simulink model "gm_commhdlQPSKTxRx"  (R2025b)
settings: Solver=VariableStepAuto  StartTime=0.0  StopTime=10.0  RelTol=1e-3
PostLoadFcn:
  | hScopeConfig = get_param([gcs '/Receiver/QPSK Rx/Frequency and Time Synchronizer/Symbol Synchronizer/No HDL/QPSK Receiver Eye Diagram'],'ScopeConfiguration');
  | 
  | hScopeConfig.OpenAtSimulationStart = false;
  | hScopeConfig.Visible = false;
  | SamplesPerSymbol = 4;
  | %UpsamplesRx = 1;
  | clear hScopeConfig
InitFcn:
  | commhdlQPSKTxRxModelInit;
  | % Rate bridge: ADRV9002/Jupiter radio runs at 15.36 MHz = 2x the 7.68 MHz
  | % (4 samples/symbol @ Rsym=1.92 MHz) the QPSK Rx requires. The deployed
  | % Receiver must downsample the ADC stream by 2. UpsamplesRx=1 fed the QPSK
  | % Rx 8 sps (2x-upsampled) and broke symbol sync / the loopback bit check.
  | UpsamplesRx = 2;
  | UpsamplesTx = 1;
  | clear simTimingOffset;
StopFcn:
  | if exist('simTimingOffset','var')
  |   disp('Simulation completed');
  |   %QPSKTxRxVerification;
  | end
undefined symbols (not defined in the file or in its folder): Add, Config, Error, fsym, Ignore, randsrc, RandStream, Rsym, Shift
libraries: hdlsllib x64, dspsigops x19, simulink x19, dsphdlfiltering2 x3, dsphdlsigops2 x2, dsphdlmathfun2 x2, commdigbbndpm3 x2, commchan3 x1, commrflib2 x1
(part 8 of 9)

== system gm_commhdlQPSKTxRx/Receiver/QPSK Rx/Frequency and Time Synchronizer/Phase Ambiguity Estimation and Correction/Phase Ambiguity Estimator ==
  dataIn : Inport  OutDataTypeStr=fixdt(1, 16, 14)  PortDimensions=1  SampleTime=1.30208333333333e-07
      settings: SignalType=complex
  syncPulse : Inport  Port=2  OutDataTypeStr=boolean  PortDimensions=1  SampleTime=1.30208333333333e-07
  validIn : Inport  Port=3  OutDataTypeStr=boolean  PortDimensions=1  SampleTime=1.30208333333333e-07
  Compare To Constant : simulink/Logic and Bit Operations/Compare To Constant  relop===  const=7  OutDataTypeStr=boolean
  Delay{1..3,8} (4 alike) : Delay  DelayLength=1
  Delay{4..7,9..11} (7 alike) : Delay
  Direct Lookup Table (n-D) : LookupNDDirect  NumberOfTableDimensions=1  Table=fi(preambleSymbols(3+1:3+8),1,16)  DiagnosticForOutOfRangeInput=Error
  HDL Counter : hdlsllib/Sources/HDL Counter  CountType=Count limited  CountInit=0  CountStep=1  CountMax=8-1  CountFromType=Initial value  CountFrom=0  CountResetPort=on  CountLoadPort=off  CountEnbPort=on  CountDirPort=off  CountHitOutputPort=off  CountDataType=Unsigned  CountWordLen=3  CountFracLen=0  CountSampTime=1
  Logical Operator : Logic  IconShape=distinctive  AllPortsSameDT=off  OutDataTypeStr=boolean
  Math Function : Math  Operator=conj  SignedPower=on  OutDataTypeStr=fixdt(1, 16, 15)  RndMeth=Zero
  Product : Product  OutDataTypeStr=fixdt(1, 32, 29)
  Subsystem : Subsystem
  Subsystem1 : Subsystem
  endOut : Outport  SampleTime=1.30208333333333e-07
  estOut : Outport  Port=2  SampleTime=1.30208333333333e-07
  validOut : Outport  Port=3  SampleTime=1.30208333333333e-07
  wires:
  Product/1 -> Delay9/1
  Delay11/1 -> endOut/1
  Delay5/1 -> Product/1
  Math Function/1 -> Delay4/1
  Delay1/1 -> Delay5/1
  Subsystem1/1(validOut) -> Delay2/1, Logical Operator/1, HDL Counter/2
  validIn/1 -> Subsystem1/2(validIn)
  Delay2/1 -> Delay6/1
  Subsystem/1(Out2) -> HDL Counter/1, Subsystem1/1(In1)
  Logical Operator/1 -> Delay3/1, Subsystem/2(H)
  Delay6/1 -> Delay10/1
  HDL Counter/1 -> Delay8/1, Compare To Constant/1
  Delay9/1 -> estOut/1
  Compare To Constant/1 -> Logical Operator/2
  Delay4/1 -> Product/2
  Delay10/1 -> validOut/1
  Delay3/1 -> Delay7/1
  syncPulse/1 -> Subsystem/1(L)
  Delay8/1 -> Direct Lookup Table (n-D)/1
  Delay7/1 -> Delay11/1
  dataIn/1 -> Delay1/1
  Direct Lookup Table (n-D)/1 -> Math Function/1

== system gm_commhdlQPSKTxRx/Receiver/QPSK Rx/Frequency and Time Synchronizer/Preamble Detector/Correlator ==
  dataIn : Inport  OutDataTypeStr=fixdt(1, 16, 14)  PortDimensions=1  SampleTime=1.30208333333333e-07
      settings: SignalType=complex
  validIn : Inport  Port=2  OutDataTypeStr=boolean  PortDimensions=1  SampleTime=1.30208333333333e-07
  Complex to Real-Imag : ComplexToRealImag  Output=Real
  Delay{1..6} (6 alike) : Delay  DelayLength=1
  Delay7 : Delay  DelayLength=4
  Delay8 : Delay  DelayLength=4
  Discrete FIR Filter : dsphdlfiltering2/Discrete FIR Filter  NumeratorSource=Property  Numerator=rxPreambleMFCoeffs  NumeratorPrototype=[]  FilterStructure=Direct form systolic  SerializationOption=Minimum number of cycles between valid input samples  NumCycles=2  NumberOfMultipliers=2  SimulateUsing=Code generation  roundingMode=Floor  overflowMode=off  CoefficientsDataTypeStr=Inherit: Same word length as input  OutputDataTypeStr=Inherit: Same word length as input  ResetInputPort=off  HDLGlobalReset=off  CoeffMultiplier=Multiplier  UseMultForPow2Coeff=on  FrameInputSymmOptim=off
  Magnitude Squared : Subsystem
  Magnitude Squared and Moving Sum : Subsystem
  ThresholdLimiter : Subsystem
  dataOut : Outport  SampleTime=1.30208333333333e-07
  threshold : Outport  Port=2  SampleTime=1.30208333333333e-07
  validOut : Outport  Port=3  SampleTime=1.30208333333333e-07
  wires:
  Delay2/1 -> dataOut/1
  Delay5/1 -> threshold/1
  Delay8/1 -> Delay5/1
  Delay7/1 -> Delay3/1
  validIn/1 -> Discrete FIR Filter/2, Magnitude Squared and Moving Sum/2(validIn)
  ThresholdLimiter/1(y) -> Delay8/1
  Discrete FIR Filter/1 -> Delay6/1
  Delay6/1 -> Magnitude Squared/1(In1)
  dataIn/1 -> Discrete FIR Filter/1, Magnitude Squared and Moving Sum/1(scaled1)
  Delay3/1 -> validOut/1
  Magnitude Squared and Moving Sum/1(E1) -> Delay4/1
  Discrete FIR Filter/2 -> Delay1/1
  Delay1/1 -> Delay7/1
  Delay4/1 -> ThresholdLimiter/1(x)
  Magnitude Squared/1(Out1) -> Complex to Real-Imag/1
  Complex to Real-Imag/1 -> Delay2/1

== system gm_commhdlQPSKTxRx/Receiver/QPSK Rx/Frequency and Time Synchronizer/Preamble Detector/FIFO ==
  in : Inport  OutDataTypeStr=fixdt(1, 16, 14)  PortDimensions=1  SampleTime=1.30208333333333e-07
      settings: SignalType=complex
  push : Inport  Port=2  OutDataTypeStr=boolean  PortDimensions=1  SampleTime=1.30208333333333e-07
  pop : Inport  Port=3  OutDataTypeStr=boolean  PortDimensions=1  SampleTime=1.30208333333333e-07
  reset : Inport  Port=4  OutDataTypeStr=boolean  PortDimensions=1  SampleTime=1.30208333333333e-07
  Delay1 : Delay  DelayLength=1
  Pop Counter : hdlsllib/Sources/HDL Counter  CountType=Count limited  CountInit=0  CountStep=1  CountMax=fifoSize -1  CountFromType=Initial value  CountFrom=0  CountResetPort=on  CountLoadPort=off  CountEnbPort=on  CountDirPort=off  CountHitOutputPort=off  CountDataType=Unsigned  CountWordLen=nextpow2(fifoSize)  CountFracLen=0  CountSampTime=1
  Push Counter : hdlsllib/Sources/HDL Counter  CountType=Count limited  CountInit=0  CountStep=1  CountMax=fifoSize -1  CountFromType=Initial value  CountFrom=0  CountResetPort=on  CountLoadPort=off  CountEnbPort=on  CountDirPort=off  CountHitOutputPort=off  CountDataType=Unsigned  CountWordLen=nextpow2(fifoSize)  CountFracLen=0  CountSampTime=1
  Simple Dual Port RAM : hdlsllib/HDL RAMs/Simple Dual Port RAM  ram_size=nextpow2(fifoSize)
  Validate Input Push Pop : Subsystem
  out : Outport  SampleTime=1.30208333333333e-07
  wires:
  Simple Dual Port RAM/1 -> out/1
  Pop Counter/1 -> Simple Dual Port RAM/4
  Push Counter/1 -> Simple Dual Port RAM/2
  in/1 -> Simple Dual Port RAM/1
  Delay1/1 -> Push Counter/1, Pop Counter/1
  pop/1 -> Validate Input Push Pop/3(pop)
  Validate Input Push Pop/2(valid pop) -> Pop Counter/2
  Validate Input Push Pop/1(valid push) -> Push Counter/2, Simple Dual Port RAM/3
  push/1 -> Validate Input Push Pop/2(push)
  reset/1 -> Validate Input Push Pop/1(rst), Delay1/1

== system gm_commhdlQPSKTxRx/Receiver/QPSK Rx/Frequency and Time Synchronizer/Preamble Detector/Peak Search ==
  note: peak picker
  corr : Inport  OutDataTypeStr=fixdt(1, 32, 26)  PortDimensions=1  SampleTime=1.30208333333333e-07
  thresholdExceeded : Inport  Port=2  OutDataTypeStr=boolean  PortDimensions=1  SampleTime=1.30208333333333e-07
  validIn : Inport  Port=3  OutDataTypeStr=boolean  PortDimensions=1  SampleTime=1.30208333333333e-07
  Compare To Constant : simulink/Logic and Bit Operations/Compare To Constant  relop===  const=samplesPerFrame1x - 1  OutDataTypeStr=boolean
  Logical Operator : Logic  IconShape=distinctive  AllPortsSameDT=off  OutDataTypeStr=boolean
  Logical Operator4 : Logic  IconShape=distinctive  AllPortsSameDT=off  OutDataTypeStr=boolean
  Relational Operator : RelationalOperator  Operator=>  OutDataTypeStr=boolean  InputSameDT=off
  Unit Delay Enabled Resettable Synchronous : hdlsllib/Discrete/Unit Delay Enabled Resettable Synchronous  InitialCondition=0.0  SampleTime=-1
  Unit Delay Enabled Resettable Synchronous1 : hdlsllib/Discrete/Unit Delay Enabled Resettable Synchronous  InitialCondition=0.0  SampleTime=-1
  Unit Delay Enabled Synchronous : hdlsllib/Discrete/Unit Delay Enabled Synchronous  InitialCondition=0.0  SampleTime=-1
  timing Reference : hdlsllib/Sources/HDL Counter  CountType=Count limited  CountInit=0  CountStep=1  CountMax=samplesPerFrame1x - 1  CountFromType=Initial value  CountFrom=0  CountResetPort=off  CountLoadPort=off  CountEnbPort=on  CountDirPort=off  CountHitOutputPort=off  CountDataType=Unsigned  CountWordLen=nextpow2(samplesPerFrame1x - 1)  CountFracLen=0  CountSampTime=1
  timingOffset : Outport  SampleTime=1.30208333333333e-07
  done : Outport  Port=2  SampleTime=1.30208333333333e-07
  success : Outport  Port=3  SampleTime=1.30208333333333e-07
  wires:
  Unit Delay Enabled Synchronous/1 -> timingOffset/1
  Logical Operator4/1 -> Unit Delay Enabled Synchronous/2, Unit Delay Enabled Resettable Synchronous/2
  Relational Operator/1 -> Logical Operator4/1
  Unit Delay Enabled Resettable Synchronous1/1 -> success/1
  Unit Delay Enabled Resettable Synchronous/1 -> Relational Operator/2
  corr/1 -> Unit Delay Enabled Resettable Synchronous/1, Relational Operator/1
  thresholdExceeded/1 -> Unit Delay Enabled Resettable Synchronous1/1, Unit Delay Enabled Resettable Synchronous1/2, Logical Operator4/2
  Logical Operator/1 -> done/1, Unit Delay Enabled Resettable Synchronous/3, Unit Delay Enabled Resettable Synchronous1/3
  Compare To Constant/1 -> Logical Operator/2
  timing Reference/1 -> Compare To Constant/1, Unit Delay Enabled Synchronous/1
  validIn/1 -> timing Reference/1, Logical Operator/1

== system gm_commhdlQPSKTxRx/Receiver/QPSK Rx/Frequency and Time Synchronizer/Preamble Detector/Timing Adjust ==
  timingOffset : Inport  OutDataTypeStr=fixdt(0, 11, 0)  PortDimensions=1  SampleTime=1.30208333333333e-07
  timingOffsetValid : Inport  Port=2  OutDataTypeStr=boolean  PortDimensions=1  SampleTime=1.30208333333333e-07
  dataIn : Inport  Port=3  OutDataTypeStr=fixdt(1, 16, 14)  PortDimensions=1  SampleTime=1.30208333333333e-07
      settings: SignalType=complex
  validIn : Inport  Port=4  OutDataTypeStr=boolean  PortDimensions=1  SampleTime=1.30208333333333e-07
  Delay{,1..4} (5 alike) : Delay  DelayLength=1
  Logical Operator : Logic  AllPortsSameDT=off  OutDataTypeStr=boolean
  Logical Operator1 : Logic  Operator=NOT  AllPortsSameDT=off  OutDataTypeStr=boolean
  Logical Operator2 : Logic  Inputs=3  AllPortsSameDT=off  OutDataTypeStr=boolean
  Relational Operator : RelationalOperator  Operator===  OutDataTypeStr=boolean  InputSameDT=off
  State Register : hdlsllib/Discrete/Unit Delay Enabled Resettable Synchronous  InitialCondition=0.0  SampleTime=-1
  Unit Delay Enabled Synchronous3 : hdlsllib/Discrete/Unit Delay Enabled Synchronous  InitialCondition=0.0  SampleTime=-1
  timing Reference : hdlsllib/Sources/HDL Counter  CountType=Count limited  CountInit=0  CountStep=1  CountMax=searchSamples - 1  CountFromType=Initial value  CountFrom=0  CountResetPort=off  CountLoadPort=off  CountEnbPort=on  CountDirPort=off  CountHitOutputPort=off  CountDataType=Unsigned  CountWordLen=nextpow2(searchSamples - 1)  CountFracLen=0  CountSampTime=1
  dataOut : Outport  SampleTime=1.30208333333333e-07
  validOut : Outport  Port=2  SampleTime=1.30208333333333e-07
  SyncPulse : Outport  Port=3  SampleTime=1.30208333333333e-07
  wires:
  Delay/1 -> SyncPulse/1
  Logical Operator2/1 -> Delay/1, Delay2/1
  timingOffsetValid/1 -> Logical Operator/1
  dataIn/1 -> Delay4/1
  Logical Operator1/1 -> Logical Operator/2
  Delay4/1 -> dataOut/1
  validIn/1 -> timing Reference/1, Delay3/1, Logical Operator2/1
  timingOffset/1 -> Unit Delay Enabled Synchronous3/1
  Logical Operator/1 -> State Register/1, State Register/2, Unit Delay Enabled Synchronous3/2
  Delay3/1 -> validOut/1
  Unit Delay Enabled Synchronous3/1 -> Relational Operator/2
  timing Reference/1 -> Relational Operator/1
  Relational Operator/1 -> Logical Operator2/2
  State Register/1 -> Logical Operator2/3, Delay1/1
  Delay1/1 -> Logical Operator1/1
  Delay2/1 -> State Register/3

== system gm_commhdlQPSKTxRx/Receiver/QPSK Rx/Frequency and Time Synchronizer/Symbol Synchronizer/Gardner TED ==
  data : Inport  OutDataTypeStr=fixdt(1, 19, 12)  PortDimensions=1  SampleTime=1.30208333333333e-07
      settings: SignalType=complex
  strobe : Inport  Port=2  OutDataTypeStr=boolean  PortDimensions=1  SampleTime=1.30208333333333e-07
  Constant : Constant  Value=0  OutDataTypeStr=fixdt(1, 40, 24)  SampleTime=1/(Rsym*SamplesPerSymbol)
  Delay10 : Delay  DelayLength=4
  GTED : Subsystem
  Switch : Switch  Criteria=u2 ~= 0  OutDataTypeStr=fixdt(1, 40, 24)  InputSameDT=off
  e : Outport  SampleTime=1.30208333333333e-07  VectorParamsAs1DForOutWhenUnconnected=off
  wires:
  Switch/1 -> e/1
  Delay10/1 -> Switch/2
  GTED/1(Out1) -> Switch/1
  strobe/1 -> Delay10/1
  Constant/1 -> Switch/3
  data/1 -> GTED/1(In1)

== system gm_commhdlQPSKTxRx/Receiver/QPSK Rx/Frequency and Time Synchronizer/Symbol Synchronizer/Interpolation Control ==
  Delta : Inport  OutDataTypeStr=fixdt(1, 11, 10)  PortDimensions=1  SampleTime=1.30208333333333e-07
  Interpolation Control : MATLAB Function
  mu : Outport  SampleTime=1.30208333333333e-07
  Underflow : Outport  Port=2  SampleTime=1.30208333333333e-07
  wires:
  Delta/1 -> Interpolation Control/1(Delta)
  Interpolation Control/1(mu) -> mu/1
  Interpolation Control/2(Underflow) -> Underflow/1

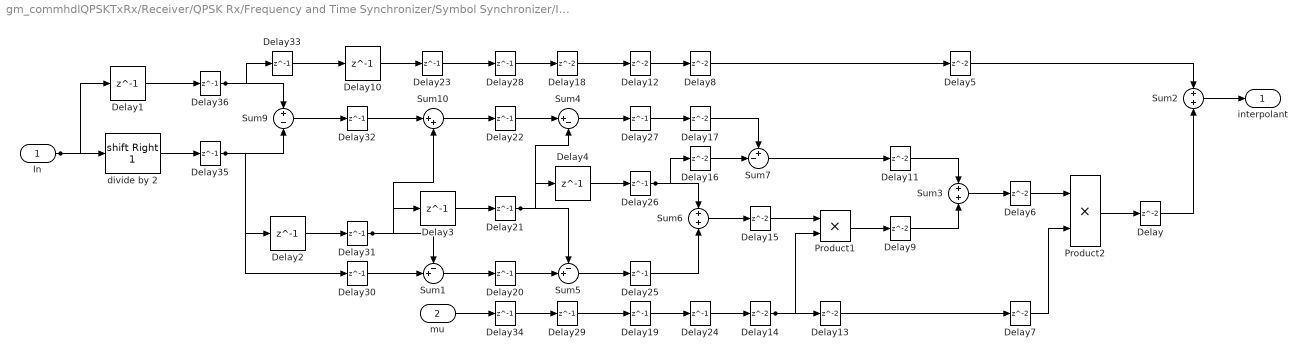
== system gm_commhdlQPSKTxRx/Receiver/QPSK Rx/Frequency and Time Synchronizer/Symbol Synchronizer/Interpolation Filter ==
  In : Inport  OutDataTypeStr=fixdt(1, 16, 12)  PortDimensions=1  SampleTime=1.30208333333333e-07
      settings: SignalType=complex
  mu : Inport  Port=2  OutDataTypeStr=fixdt(1, 11, 10)  PortDimensions=1  SampleTime=1.30208333333333e-07
  Delay{,5..9,11..18} (14 alike) : Delay
  Delay{1..4,10} (5 alike) : Delay  DelayLength=1  InitialCondition=0
  Delay{19..36} (18 alike) : Delay  DelayLength=1
  Product1 : Product  OutDataTypeStr=fixdt(1,16,10)  RndMeth=Zero
  Product2 : Product  OutDataTypeStr=fixdt(1, 16, 10)  RndMeth=Zero
  Sum1 : Sum  Inputs=-+|  OutDataTypeStr=fixdt(1, 17, 12)
  Sum10 : Sum  Inputs=|++  OutDataTypeStr=fixdt(1, 18, 12)
  Sum2 : Sum  Inputs=+|+  OutDataTypeStr=fixdt(1, 19, 12)
  Sum3 : Sum  Inputs=+|+  OutDataTypeStr=fixdt(1,16,10)
  Sum4 : Sum  Inputs=|+-  OutDataTypeStr=fixdt(1, 19, 12)
  Sum5 : Sum  Inputs=-+|  OutDataTypeStr=fixdt(1, 18, 12)
  Sum6 : Sum  Inputs=+|+  OutDataTypeStr=fixdt(1,16,11)  SaturateOnIntegerOverflow=on
  Sum7 : Sum  Inputs=+-|  OutDataTypeStr=fixdt(1,16,10)
  Sum9 : Sum  Inputs=+-  OutDataTypeStr=fixdt(1, 17, 12)
  divide by 2 : ArithShift  BitShiftNumber=1  BitShiftDirection=Right
  interpolant : Outport  SampleTime=1.30208333333333e-07
  wires:
  Delay/1 -> Sum2/2
  Product2/1 -> Delay/1
  Delay6/1 -> Product2/1
  Delay5/1 -> Sum2/1
  Delay13/1 -> Delay7/1
  Sum7/1 -> Delay11/1
  Sum3/1 -> Delay6/1
  Delay24/1 -> Delay14/1
  Delay16/1 -> Sum7/2
  Delay17/1 -> Sum7/1
  Delay8/1 -> Delay5/1
  Delay19/1 -> Delay24/1
  Delay26/1 -> Delay16/1, Sum6/1
  Delay7/1 -> Product2/2
  Delay31/1 -> Delay3/1, Sum1/1, Sum10/2
  Delay15/1 -> Product1/1
  Delay2/1 -> Delay31/1
  Delay35/1 -> Delay2/1, Delay30/1, Sum9/2
  Sum9/1 -> Delay32/1
  Delay23/1 -> Delay28/1
  Sum1/1 -> Delay20/1
  Delay33/1 -> Delay10/1
  Delay4/1 -> Delay26/1
  Delay36/1 -> Delay33/1, Sum9/1
  Delay25/1 -> Sum6/2
  Delay12/1 -> Delay8/1
  Sum5/1 -> Delay25/1
  Delay28/1 -> Delay18/1
  divide by 2/1 -> Delay35/1
  Delay1/1 -> Delay36/1
  Delay14/1 -> Delay13/1, Product1/2
  Delay3/1 -> Delay21/1
  Product1/1 -> Delay9/1
  Delay34/1 -> Delay29/1
  Delay30/1 -> Sum1/2
  Delay32/1 -> Sum10/1
  Delay10/1 -> Delay23/1
  Sum4/1 -> Delay27/1
  Sum10/1 -> Delay22/1
  Delay9/1 -> Sum3/2
  Delay21/1 -> Delay4/1, Sum4/2, Sum5/1
  Delay11/1 -> Sum3/1
  mu/1 -> Delay34/1
  Sum2/1 -> interpolant/1
  In/1 -> Delay1/1, divide by 2/1
  Delay22/1 -> Sum4/1
  Delay20/1 -> Sum5/2
  Delay18/1 -> Delay12/1
  Delay29/1 -> Delay19/1
  Sum6/1 -> Delay15/1
  Delay27/1 -> Delay17/1

== system gm_commhdlQPSKTxRx/Receiver/QPSK Rx/Frequency and Time Synchronizer/Symbol Synchronizer/Loop Filter ==
  e : Inport  OutDataTypeStr=fixdt(1, 40, 24)  PortDimensions=1  SampleTime=1.30208333333333e-07
  Add : Sum  OutDataTypeStr=fixdt(1, 31, 23)
  Add2 : Sum  Inputs=|++  OutDataTypeStr=fixdt(1, 30, 23)
  Data Type Conversion17 : DataTypeConversion  OutDataTypeStr=fixdt(1,11,10)  SaturateOnIntegerOverflow=off  RndMeth=Floor
  Delay : Delay  DelayLength=1
  Delay1 : Delay  DelayLength=1  InitialCondition=0
  Delay2 : Delay  InitialCondition=0
  Delay3 : Delay  InitialCondition=0
  Delay4 : Delay  DelayLength=1  InitialCondition=0
  Delay5 : Delay  InitialCondition=0
  Delay6 : Delay  DelayLength=1
  K1 : Gain  Gain=fi(SSLoopFilterPropGain,1,24,24)  ParamDataTypeStr=Inherit: Inherit from 'Gain'  OutDataTypeStr=fixdt(1,30,23)
  K2 : Gain  Gain=fi(SSLoopFilterIntegGain,1,24,24)  ParamDataTypeStr=Inherit: Inherit from 'Gain'  OutDataTypeStr=fixdt(1,30,23)
  v : Outport  SampleTime=1.30208333333333e-07
  wires:
  Add2/1 -> Delay4/1, Delay/1
  Delay6/1 -> Add2/1
  Add/1 -> Data Type Conversion17/1
  Delay/1 -> Add2/2
  Delay5/1 -> Delay6/1
  Data Type Conversion17/1 -> v/1
  Delay4/1 -> Add/2
  Delay3/1 -> Delay1/1
  K2/1 -> Delay5/1
  K1/1 -> Delay3/1
  Delay1/1 -> Add/1
  Delay2/1 -> K1/1, K2/1
  e/1 -> Delay2/1

== system gm_commhdlQPSKTxRx/Receiver/QPSK Rx/Frequency and Time Synchronizer/Symbol Synchronizer/Rate Handle ==
  dataIn : Inport  OutDataTypeStr=fixdt(1, 16, 14)  PortDimensions=1  SampleTime=1.30208333333333e-07
      settings: SignalType=complex
  strobe : Inport  Port=2  OutDataTypeStr=boolean  PortDimensions=1  SampleTime=1.30208333333333e-07
  validIn : Inport  Port=3  OutDataTypeStr=boolean  PortDimensions=1  SampleTime=1.30208333333333e-07
  Compare To Constant : simulink/Logic and Bit Operations/Compare To Constant  relop===  const=0  OutDataTypeStr=boolean
  Constant : Constant  Value=false  OutDataTypeStr=boolean  SampleTime=-1
  FIFO : Subsystem  mask{fifoSize=double(32), pushFullDiag=Error, popEmptyDiag=Ignore}
      mask prompts: fifoSize "FIFO size:"; pushFullDiag "Push full FIFO:"; popEmptyDiag "Pop empty FIFO:"
      mask TypeOptions pushFullDiag: Ignore | Warning | Error
      mask TypeOptions popEmptyDiag: Ignore | Warning | Error
  HDL Counter : hdlsllib/Sources/HDL Counter  CountType=Count limited  CountInit=0  CountStep=1  CountMax=SamplesPerSymbol - 1  CountFromType=Initial value  CountFrom=0  CountResetPort=off  CountLoadPort=off  CountEnbPort=on  CountDirPort=off  CountHitOutputPort=off  CountDataType=Unsigned  CountWordLen=nextpow2(SamplesPerSymbol - 1)  CountFracLen=0  CountSampTime=1
  Logical Operator : Logic  AllPortsSameDT=off  OutDataTypeStr=boolean
  dataOut : Outport  SampleTime=1.30208333333333e-07
  validOut : Outport  Port=2  SampleTime=1.30208333333333e-07
  wires:
  FIFO/2(validPop) -> validOut/1
  FIFO/1(out) -> dataOut/1
  strobe/1 -> FIFO/2(push)
  dataIn/1 -> FIFO/1(in)
  Logical Operator/1 -> FIFO/3(pop)
  Compare To Constant/1 -> Logical Operator/2
  Constant/1 -> FIFO/4(reset)
  HDL Counter/1 -> Compare To Constant/1
  validIn/1 -> HDL Counter/1, Logical Operator/1

== system gm_commhdlQPSKTxRx/Transmitter/QPSK Tx/Bit Packetizer/Data Bits FIFO/No HDL ==
  push : Inport
  pop : Inport  Port=2
  MATLAB Function : MATLAB Function  TreatAsAtomicUnit=on
  No HDL : Subsystem
  wires:
  MATLAB Function/3(empty) -> No HDL/4(empty)
  MATLAB Function/1(full) -> No HDL/2(full)
  MATLAB Function/2(ncount) -> No HDL/3(ncount)
  pop/1 -> No HDL/5(pop), MATLAB Function/2(rd)
  push/1 -> No HDL/1(push), MATLAB Function/1(wr)

== system gm_commhdlQPSKTxRx/Transmitter/QPSK Tx/Bit Packetizer/Preamble Bits Generator/Preamble Bits Store ==
  note: The Preamble is padded with zeros in the LUT such that
      | the length is the 2^nextpow2(length(Preamble)) for
      | efficient resource mapping to RAM
  actualPreamble : Inport
  sampleCount : Inport  Port=2
  Constant : Constant  OutDataTypeStr=boolean  SampleTime=1/(Rsym*4)
  Extract Bits : simulink/Logic and Bit Operations/Extract Bits  bitsToExtract=Range of bits  numBits=8  bitIdxRange=[0 nextpow2(length(Preamble))-1]  outScalingMode=Treat bit field as an integer
  Preamble : LookupNDDirect  NumberOfTableDimensions=1  Table=[Preamble;false(32-length(Preamble),1)]  DiagnosticForOutOfRangeInput=Error
  Switch : Switch  Criteria=u2 ~= 0  Threshold=1  SaturateOnIntegerOverflow=off  InputSameDT=off
  preamble : Outport
  wires:
  actualPreamble/1 -> Switch/2
  sampleCount/1 -> Extract Bits/1
  Preamble/1 -> Switch/1
  Extract Bits/1 -> Preamble/1
  Constant/1 -> Switch/3
  Switch/1 -> preamble/1

== system gm_commhdlQPSKTxRx/Receiver/QPSK Rx/Frequency and Time Synchronizer/Coarse Frequency Compensator/Coarse Frequency Estimator/Extract Frequency ==
  datain : Inport  OutDataTypeStr=fixdt(1, 32, 24)  PortDimensions=1  SampleTime=1.30208333333333e-07
      settings: SignalType=complex
  validIn : Inport  Port=2  OutDataTypeStr=boolean  PortDimensions=1  SampleTime=1.30208333333333e-07
  Complex to Magnitude-Angle HDL Optimized : dsphdlmathfun2/Complex to Magnitude-Angle  NumIterationsSource=Auto  NumIterations=10  OutputFormat=Angle  AngleFormat=Normalized  ScaleOutput=on  ScalingMethod=Shift-Add  SimulateUsing=Code generation
  Delay{1..4} (4 alike) : Delay  DelayLength=1
  Gain : Gain  Gain=1/2  ParamDataTypeStr=fixdt(0,1,1)  OutDataTypeStr=fixdt(1, 35, 34)
  Unit Delay Enabled Synchronous : hdlsllib/Discrete/Unit Delay Enabled Synchronous  InitialCondition=0.0  SampleTime=-1
  normFreqOut : Outport  SampleTime=1.30208333333333e-07
  wires:
  Delay3/1 -> normFreqOut/1
  Gain/1 -> Delay3/1
  Delay2/1 -> Gain/1
  Unit Delay Enabled Synchronous/1 -> Delay2/1
  Complex to Magnitude-Angle HDL Optimized/2 -> Unit Delay Enabled Synchronous/2
  Complex to Magnitude-Angle HDL Optimized/1 -> Unit Delay Enabled Synchronous/1
  Delay4/1 -> Complex to Magnitude-Angle HDL Optimized/2
  Delay1/1 -> Complex to Magnitude-Angle HDL Optimized/1
  validIn/1 -> Delay4/1
  datain/1 -> Delay1/1

== system gm_commhdlQPSKTxRx/Receiver/QPSK Rx/Frequency and Time Synchronizer/Coarse Frequency Compensator/Coarse Frequency Estimator/Integrator ==
  note: store the value in the Reg before reset
  dataIn : Inport  OutDataTypeStr=fixdt(1, 32, 24)  PortDimensions=1  SampleTime=1.30208333333333e-07
      settings: SignalType=complex
  validIn : Inport  Port=2  OutDataTypeStr=boolean  PortDimensions=1  SampleTime=1.30208333333333e-07
  Add1 : Sum  Inputs=|++  OutDataTypeStr=fixdt(1, 32, 24)
  Delay : Delay  DelayLength=1
  Delay1 : Delay  DelayLength=1
  Delay2 : Delay  DelayLength=1
  Integ Reg : hdlsllib/Discrete/Unit Delay Enabled Resettable Synchronous  InitialCondition=0.0  SampleTime=-1
  Reset Generator : Subsystem
  Store Reg : hdlsllib/Discrete/Unit Delay Enabled Synchronous  InitialCondition=0.0  SampleTime=-1
  IntegOut : Outport  SampleTime=1.30208333333333e-07
  IntegValid : Outport  Port=2  SampleTime=1.30208333333333e-07
  wires:
  Add1/1 -> Integ Reg/1
  Integ Reg/1 -> Store Reg/1, Add1/2
  Delay1/1 -> Add1/1
  Delay/1 -> IntegValid/1
  Delay2/1 -> Integ Reg/2
  dataIn/1 -> Delay1/1
  Store Reg/1 -> IntegOut/1
  Reset Generator/1(reset) -> Delay/1, Integ Reg/3, Store Reg/2
  validIn/1 -> Reset Generator/1(validIn), Delay2/1

== system gm_commhdlQPSKTxRx/Receiver/QPSK Rx/Frequency and Time Synchronizer/Phase Ambiguity Estimation and Correction/Phase Ambiguity Corrector/Reciprocal ==
  dataIn : Inport  OutDataTypeStr=fixdt(1, 13, 10)  PortDimensions=1  SampleTime=1.30208333333333e-07
  Compare To Constant : simulink/Logic and Bit Operations/Compare To Constant  relop=<  const=0  OutDataTypeStr=boolean
  Data Type Conversion : DataTypeConversion  OutDataTypeStr=fixdt(1,WL,0)  ConvertRealWorld=Stored Integer (SI)  SaturateOnIntegerOverflow=off  RndMeth=Floor
  Data Type Conversion1 : DataTypeConversion  OutDataTypeStr=fixdt(0,LUTAddrWL,0)  ConvertRealWorld=Stored Integer (SI)  SaturateOnIntegerOverflow=off  RndMeth=Floor
  Data Type Conversion2 : DataTypeConversion  OutDataTypeStr=fixdt(0,WL-LUTAddrWL,0)  ConvertRealWorld=Stored Integer (SI)  SaturateOnIntegerOverflow=off  RndMeth=Floor
  Delay : Delay  DelayLength=1
  Delay1 : Delay  DelayLength=1
  Delay2 : Delay  DelayLength=1
  Extract Bits : simulink/Logic and Bit Operations/Extract Bits  bitsToExtract=Range ending with least significant bit  numBits=LUTAddrWL  bitIdxRange=[0 7]  outScalingMode=Treat bit field as an integer
  Function Impl : Subsystem
  dataOut : Outport  SampleTime=1.30208333333333e-07
  wires:
  Function Impl/1(functionValues) -> dataOut/1
  Data Type Conversion2/1 -> Function Impl/1(switch)
  Data Type Conversion1/1 -> Function Impl/2(LUTAddr)
  Delay1/1 -> Data Type Conversion2/1
  Compare To Constant/1 -> Delay1/1
  Delay2/1 -> Data Type Conversion1/1
  Extract Bits/1 -> Delay2/1
  Delay/1 -> Compare To Constant/1, Extract Bits/1
  Data Type Conversion/1 -> Delay/1
  dataIn/1 -> Data Type Conversion/1

== system gm_commhdlQPSKTxRx/Receiver/QPSK Rx/Frequency and Time Synchronizer/Phase Ambiguity Estimation and Correction/Phase Ambiguity Estimator/Subsystem ==
  L : Inport  OutDataTypeStr=boolean  PortDimensions=1  SampleTime=1.30208333333333e-07
  H : Inport  Port=2  OutDataTypeStr=boolean  PortDimensions=1  SampleTime=1.30208333333333e-07
  Delay6 : Delay  DelayLength=1  InitialCondition=1
  Logical Operator : Logic  AllPortsSameDT=off  OutDataTypeStr=boolean
  Logical Operator1 : Logic  Operator=NOT  IconShape=distinctive  AllPortsSameDT=off  OutDataTypeStr=boolean
  Logical Operator2 : Logic  Operator=OR  AllPortsSameDT=off  OutDataTypeStr=boolean
  Out2 : Outport  SampleTime=1.30208333333333e-07
  wires:
  Logical Operator/1 -> Logical Operator2/2
  Delay6/1 -> Out2/1, Logical Operator/2
  Logical Operator1/1 -> Logical Operator/1
  Logical Operator2/1 -> Delay6/1
  L/1 -> Logical Operator1/1
  H/1 -> Logical Operator2/1

== system gm_commhdlQPSKTxRx/Receiver/QPSK Rx/Frequency and Time Synchronizer/Phase Ambiguity Estimation and Correction/Phase Ambiguity Estimator/Subsystem1 ==
  In1 : Inport  OutDataTypeStr=boolean  PortDimensions=1  SampleTime=1.30208333333333e-07
  validIn : Inport  Port=2  OutDataTypeStr=boolean  PortDimensions=1  SampleTime=1.30208333333333e-07
  Logical Operator1 : Logic  IconShape=distinctive  AllPortsSameDT=off  OutDataTypeStr=boolean
  Logical Operator2 : Logic  Operator=NOT  IconShape=distinctive  AllPortsSameDT=off  OutDataTypeStr=boolean
  validOut : Outport  SampleTime=1.30208333333333e-07
  wires:
  Logical Operator1/1 -> validOut/1
  validIn/1 -> Logical Operator1/2
  Logical Operator2/1 -> Logical Operator1/1
  In1/1 -> Logical Operator2/1

== system gm_commhdlQPSKTxRx/Receiver/QPSK Rx/Frequency and Time Synchronizer/Preamble Detector/Correlator/Magnitude Squared ==
  In1 : Inport  OutDataTypeStr=fixdt(1, 16, 13)  PortDimensions=1  SampleTime=1.30208333333333e-07
      settings: SignalType=complex
  Delay1 : Delay
  Delay2 : Delay
  Delay3 : Delay
  Math Function : Math  Operator=conj  OutDataTypeStr=fixdt(1, 16, 13)
  Product : Product  OutDataTypeStr=fixdt(1, 32, 26)
  Out1 : Outport  SampleTime=1.30208333333333e-07
  wires:
  Delay1/1 -> Product/2
  Delay2/1 -> Product/1
  Math Function/1 -> Delay1/1
  Delay3/1 -> Out1/1
  Product/1 -> Delay3/1
  In1/1 -> Math Function/1, Delay2/1

== system gm_commhdlQPSKTxRx/Receiver/QPSK Rx/Frequency and Time Synchronizer/Preamble Detector/Correlator/Magnitude Squared and Moving Sum ==
  scaled1 : Inport  OutDataTypeStr=fixdt(1, 16, 14)  PortDimensions=1  SampleTime=1.30208333333333e-07
      settings: SignalType=complex
  validIn : Inport  Port=2  OutDataTypeStr=boolean  PortDimensions=1  SampleTime=1.30208333333333e-07
  Add : Sum  Inputs=|+-  OutDataTypeStr=fixdt(1, 32, 28)
  Add1 : Sum  Inputs=|++  OutDataTypeStr=fixdt(1, 32, 28)
  Complex to Real-Imag1 : ComplexToRealImag  Output=Real
  Delay : Delay  DelayLength=13  ShowEnablePort=on
      settings: InputPortMap=u0,e6
  Delay{1..4,6,8..10,12} (9 alike) : Delay
  Delay11 : Delay  DelayLength=11
  Delay14 : Delay  DelayLength=1  ShowEnablePort=on
      settings: InputPortMap=u0,e6
  Delay5 : Delay  DelayLength=1
  Delay7 : Delay  DelayLength=1
  Gain : Gain  Gain=ThresoldGainFac  OutDataTypeStr=fixdt(1, 32, 28)
  Math Function1 : Math  Operator=conj  OutDataTypeStr=fixdt(1, 16, 14)
  Product1 : Product  OutDataTypeStr=fixdt(1, 32, 28)
  E1 : Outport  SampleTime=1.30208333333333e-07
  wires:
  Delay5/1 -> Add1/1
  Add/1 -> Delay5/1
  Delay/1 -> Add/2
  Delay8/1 -> Delay/2, Delay7/1
  Delay11/1 -> E1/1
  Delay7/1 -> Delay14/2
  Delay4/1 -> Delay/1, Add/1
  scaled1/1 -> Math Function1/1, Delay6/1
  Delay6/1 -> Product1/1
  Delay14/1 -> Add1/2
  Delay3/1 -> Gain/1
  Product1/1 -> Delay2/1
  Delay1/1 -> Product1/2
  Complex to Real-Imag1/1 -> Delay3/1
  Delay2/1 -> Complex to Real-Imag1/1
  Delay12/1 -> Delay10/1
  Math Function1/1 -> Delay1/1
  validIn/1 -> Delay12/1
  Delay10/1 -> Delay9/1
  Gain/1 -> Delay4/1
  Add1/1 -> Delay11/1, Delay14/1
  Delay9/1 -> Delay8/1

== system gm_commhdlQPSKTxRx/Receiver/QPSK Rx/Frequency and Time Synchronizer/Preamble Detector/Correlator/ThresholdLimiter ==
  x : Inport  OutDataTypeStr=fixdt(1, 32, 28)  PortDimensions=1  SampleTime=1.30208333333333e-07
  ThresholdLimiter : MATLAB Function  TreatAsAtomicUnit=on
  y : Outport  SampleTime=1.30208333333333e-07  VectorParamsAs1DForOutWhenUnconnected=off
  wires:
  ThresholdLimiter/1(y) -> y/1
  x/1 -> ThresholdLimiter/1(x)

== system gm_commhdlQPSKTxRx/Receiver/QPSK Rx/Frequency and Time Synchronizer/Preamble Detector/FIFO/Validate Input Push Pop ==
  rst : Inport  OutDataTypeStr=boolean  PortDimensions=1  SampleTime=1.30208333333333e-07
  push : Inport  Port=2  OutDataTypeStr=boolean  PortDimensions=1  SampleTime=1.30208333333333e-07
  pop : Inport  Port=3  OutDataTypeStr=boolean  PortDimensions=1  SampleTime=1.30208333333333e-07
  Compare To Constant : Subsystem  mask(Compare To Constant){relop===, const=double(0), OutDataTypeStr=boolean, ZeroCross=on}
      mask prompts: relop "Simulink:masks:Operator_MP"; const "Simulink:masks:ConstantValue_MP"; OutDataTypeStr "Simulink:masks:OutputDataType_MP"; ZeroCross "Simulink:masks:EnableZerocrossingDetection_MP"
      mask help: Simulink:masks:CompareToConstant_MD
      mask init:
      | OutDataTypeStr = 'boolean';
      | ZeroCross = 'on';
      | blkName = 'commhdlQPSKTxRx/Receiver/QPSK Rx/Frequency and Time Synchronizer/Preamble Detector/FIFO/Validate Input Push Pop/Compare\nTo Constant';
      | const = double(0);
      | const_str = '0';
      | const_val = double(0);
      | relop = '==';
      | setValue = 'boolean';
      | str = '== 0';
      mask TypeOptions relop: == | ~= | < | <= | >= | >
      mask TypeOptions OutDataTypeStr: Simulink:masks:uint8 | Simulink:masks:boolean
      mask Callback ZeroCross: sl('zeroCrossEnable', gcbh);
      mask Display: disp(str)
  Compare To Constant1 : Subsystem  mask(Compare To Constant){relop===, const=double(1133), OutDataTypeStr=boolean, ZeroCross=on}
      mask prompts: relop "Simulink:masks:Operator_MP"; const "Simulink:masks:ConstantValue_MP"; OutDataTypeStr "Simulink:masks:OutputDataType_MP"; ZeroCross "Simulink:masks:EnableZerocrossingDetection_MP"
      mask help: Simulink:masks:CompareToConstant_MD
      mask init:
      | OutDataTypeStr = 'boolean';
      | ZeroCross = 'on';
      | blkName = 'commhdlQPSKTxRx/Receiver/QPSK Rx/Frequency and Time Synchronizer/Preamble Detector/FIFO/Validate Input Push Pop/Compare\nTo Constant1';
      | const = double(1133);
      | const_str = 'fifoSize';
      | const_val = [];
      | relop = '==';
      | setValue = 'boolean';
      | str = '== fifoSize';
      mask TypeOptions relop: == | ~= | < | <= | >= | >
      mask TypeOptions OutDataTypeStr: Simulink:masks:uint8 | Simulink:masks:boolean
      mask Callback ZeroCross: sl('zeroCrossEnable', gcbh);
      mask Display: disp(str)
  Constant : Constant  Value=true  OutDataTypeStr=boolean  SampleTime=-1
  Constant1 : Constant  Value=false  OutDataTypeStr=boolean  SampleTime=-1
  Delay : Delay  DelayLength=1
  Logical Operator1 : Logic  Operator=XOR  AllPortsSameDT=off  OutDataTypeStr=boolean
  Logical Operator2 : Logic  Operator=NOT  AllPortsSameDT=off  OutDataTypeStr=boolean
  Logical Operator{3..5,7,9} (5 alike) : Logic  AllPortsSameDT=off  OutDataTypeStr=boolean
  Logical Operator6 : Logic  Operator=NOT  AllPortsSameDT=off  OutDataTypeStr=boolean
  Logical Operator8 : Logic  Operator=NOT  AllPortsSameDT=off  OutDataTypeStr=boolean
  MATLAB Function : Subsystem
  Switch : Switch  Criteria=u2 ~= 0  OutDataTypeStr=boolean  SaturateOnIntegerOverflow=off  InputSameDT=off
  valid push : Outport  SampleTime=1.30208333333333e-07
  valid pop : Outport  Port=2  SampleTime=1.30208333333333e-07
  wires:
  Compare To Constant1/1(y) -> Logical Operator4/2
  Compare To Constant/1(y) -> Logical Operator3/1
  Delay/1 -> Compare To Constant/1(u), Compare To Constant1/1(u)
  push/1 -> Logical Operator9/1, Logical Operator5/1
  Logical Operator6/1 -> Logical Operator7/2
  pop/1 -> Logical Operator7/1, Logical Operator3/2
  Logical Operator3/1 -> Logical Operator6/1
  Logical Operator9/1 -> valid push/1, Logical Operator1/1
  rst/1 -> MATLAB Function/1(rst)
  Constant/1 -> Switch/3
  Logical Operator8/1 -> Logical Operator5/2
  Logical Operator4/1 -> Logical Operator2/1
  Constant1/1 -> Switch/1
  Logical Operator5/1 -> Logical Operator4/1
  Logical Operator7/1 -> valid pop/1, Logical Operator1/2, Switch/2, Logical Operator8/1
  Logical Operator1/1 -> MATLAB Function/2(enb)
  Switch/1 -> MATLAB Function/3(dir)
  Logical Operator2/1 -> Logical Operator9/2
  MATLAB Function/1(count) -> Delay/1

== system gm_commhdlQPSKTxRx/Receiver/QPSK Rx/Frequency and Time Synchronizer/Symbol Synchronizer/Gardner TED/GTED ==
  In1 : Inport  OutDataTypeStr=fixdt(1, 19, 12)  PortDimensions=1  SampleTime=1.30208333333333e-07
      settings: SignalType=complex
  Add : Sum  OutDataTypeStr=fixdt(1, 40, 24)
  Add1 : Sum  Inputs=+-  OutDataTypeStr=fixdt(1, 20, 12)
  Add2 : Sum  Inputs=+-  OutDataTypeStr=fixdt(1, 20, 12)
  Complex to Real-Imag : ComplexToRealImag
  Delay{,1..7} (8 alike) : Delay  DelayLength=1
  Delay{8..13} (6 alike) : Delay
  Product : Product  OutDataTypeStr=fixdt(1, 39, 24)
  Product1 : Product  OutDataTypeStr=fixdt(1, 39, 24)
  Out1 : Outport  SampleTime=1.30208333333333e-07
  wires:
  Delay13/1 -> Add/2
  Product1/1 -> Delay13/1
  Product/1 -> Delay10/1
  Delay9/1 -> Product/2
  Add2/1 -> Delay12/1
  Complex to Real-Imag/1 -> Delay/1, Add1/2
  Complex to Real-Imag/2 -> Delay4/1, Add2/2
  Add/1 -> Out1/1
  Delay10/1 -> Add/1
  Delay6/1 -> Delay7/1
  Delay/1 -> Delay1/1
  Delay7/1 -> Add2/1
  Delay4/1 -> Delay5/1
  In1/1 -> Complex to Real-Imag/1
  Delay3/1 -> Add1/1
  Delay12/1 -> Product1/2
  Delay1/1 -> Delay2/1, Delay8/1
  Delay11/1 -> Product1/1
  Delay5/1 -> Delay6/1, Delay11/1
  Delay2/1 -> Delay3/1
  Delay8/1 -> Product/1
  Add1/1 -> Delay9/1

== system gm_commhdlQPSKTxRx/Receiver/QPSK Rx/Frequency and Time Synchronizer/Symbol Synchronizer/Rate Handle/FIFO ==
  in : Inport  OutDataTypeStr=fixdt(1, 16, 14)  PortDimensions=1  SampleTime=1.30208333333333e-07
      settings: SignalType=complex
  push : Inport  Port=2  OutDataTypeStr=boolean  PortDimensions=1  SampleTime=1.30208333333333e-07
  pop : Inport  Port=3  OutDataTypeStr=boolean  PortDimensions=1  SampleTime=1.30208333333333e-07
  reset : Inport  Port=4  OutDataTypeStr=boolean  PortDimensions=1  SampleTime=1.30208333333333e-07
  Delay1 : Delay  DelayLength=1
  Pop Counter : hdlsllib/Sources/HDL Counter  CountType=Count limited  CountInit=0  CountStep=1  CountMax=fifoSize -1  CountFromType=Initial value  CountFrom=0  CountResetPort=on  CountLoadPort=off  CountEnbPort=on  CountDirPort=off  CountHitOutputPort=off  CountDataType=Unsigned  CountWordLen=nextpow2(fifoSize)  CountFracLen=0  CountSampTime=1
  Push Counter : hdlsllib/Sources/HDL Counter  CountType=Count limited  CountInit=0  CountStep=1  CountMax=fifoSize -1  CountFromType=Initial value  CountFrom=0  CountResetPort=on  CountLoadPort=off  CountEnbPort=on  CountDirPort=off  CountHitOutputPort=off  CountDataType=Unsigned  CountWordLen=nextpow2(fifoSize)  CountFracLen=0  CountSampTime=1
  Simple Dual Port RAM : hdlsllib/HDL RAMs/Simple Dual Port RAM  ram_size=nextpow2(fifoSize)
  Validate Input Push Pop : Subsystem
  out : Outport  SampleTime=1.30208333333333e-07
  validPop : Outport  Port=2  SampleTime=1.30208333333333e-07
  wires:
  Simple Dual Port RAM/1 -> out/1
  Pop Counter/1 -> Simple Dual Port RAM/4
  Validate Input Push Pop/1(valid push) -> Push Counter/2, Simple Dual Port RAM/3
  Push Counter/1 -> Simple Dual Port RAM/2
  Delay1/1 -> Push Counter/1, Pop Counter/1
  pop/1 -> Validate Input Push Pop/3(pop)
  Validate Input Push Pop/2(valid pop) -> Pop Counter/2, validPop/1
  push/1 -> Validate Input Push Pop/2(push)
  in/1 -> Simple Dual Port RAM/1
  reset/1 -> Validate Input Push Pop/1(rst), Delay1/1

== system gm_commhdlQPSKTxRx/Transmitter/QPSK Tx/Bit Packetizer/Data Bits FIFO/No HDL/No HDL ==
  push : Inport
  full : Inport  Port=2
  ncount : Inport  Port=3
  empty : Inport  Port=4
  pop : Inport  Port=5
  Assertion : Assertion
  Assertion1 : Assertion
  Display : Display
  Logical Operator : Logic  Operator=NAND  AllPortsSameDT=off  OutDataTypeStr=boolean
  Logical Operator1 : Logic  Operator=NAND  AllPortsSameDT=off  OutDataTypeStr=boolean
  wires:
  push/1 -> Logical Operator/1
  empty/1 -> Logical Operator1/1
  full/1 -> Logical Operator/2
  pop/1 -> Logical Operator1/2
  Logical Operator/1 -> Assertion/1
  ncount/1 -> Display/1
  Logical Operator1/1 -> Assertion1/1

== system gm_commhdlQPSKTxRx/Receiver/QPSK Rx/Frequency and Time Synchronizer/Coarse Frequency Compensator/Coarse Frequency Estimator/Integrator/Reset Generator ==
  validIn : Inport  OutDataTypeStr=boolean  PortDimensions=1  SampleTime=1.30208333333333e-07
  Compare To Constant : simulink/Logic and Bit Operations/Compare To Constant  relop===  const=integAvgLen  OutDataTypeStr=boolean
  Delay1 : Delay  DelayLength=1
  Delay5 : Delay  DelayLength=1
  HDL Counter : hdlsllib/Sources/HDL Counter  CountType=Count limited  CountInit=0  CountStep=1  CountMax=integAvgLen  CountFromType=Initial value  CountFrom=0  CountResetPort=off  CountLoadPort=off  CountEnbPort=on  CountDirPort=off  CountHitOutputPort=off  CountDataType=Unsigned  CountWordLen=nextpow2(integAvgLen + 1)  CountFracLen=0  CountSampTime=1
  Logical Operator : Logic  AllPortsSameDT=off  OutDataTypeStr=boolean
  reset : Outport  SampleTime=1.30208333333333e-07
  wires:
  Logical Operator/1 -> reset/1
  Compare To Constant/1 -> Logical Operator/2
  Delay1/1 -> Logical Operator/1
  Delay5/1 -> Compare To Constant/1
  HDL Counter/1 -> Delay5/1
  validIn/1 -> HDL Counter/1, Delay1/1

== system gm_commhdlQPSKTxRx/Receiver/QPSK Rx/Frequency and Time Synchronizer/Phase Ambiguity Estimation and Correction/Phase Ambiguity Corrector/Reciprocal/Function Impl ==
  switch : Inport  OutDataTypeStr=fixdt(0, 1, 0)  PortDimensions=1  SampleTime=1.30208333333333e-07
  LUTAddr : Inport  Port=2  OutDataTypeStr=fixdt(0, 12, 0)  PortDimensions=1  SampleTime=1.30208333333333e-07
  Delay{6..8,10,15..16} (6 alike) : Delay
  Delay9 : Delay  DelayLength=1
  LUT1 : LookupNDDirect  NumberOfTableDimensions=1  Table=LUT(:,1)  DiagnosticForOutOfRangeInput=Error
  LUT2 : LookupNDDirect  NumberOfTableDimensions=1  Table=LUT(:,2)  DiagnosticForOutOfRangeInput=Error
  Multiport Switch : MultiPortSwitch  DataPortOrder=Zero-based contiguous  Inputs=2  zeroidx=on  OutDataTypeStr=fixdt(1, 26, 14)  SaturateOnIntegerOverflow=off  InputSameDT=off
  functionValues : Outport  SampleTime=1.30208333333333e-07
  wires:
  Delay16/1 -> Multiport Switch/3
  Delay15/1 -> Multiport Switch/2
  LUT1/1 -> Delay16/1
  Multiport Switch/1 -> Delay9/1
  LUT2/1 -> Delay15/1
  Delay9/1 -> functionValues/1
  Delay8/1 -> Delay10/1
  Delay6/1 -> LUT1/1
  Delay7/1 -> LUT2/1
  Delay10/1 -> Multiport Switch/1
  switch/1 -> Delay8/1
  LUTAddr/1 -> Delay6/1, Delay7/1

== system gm_commhdlQPSKTxRx/Receiver/QPSK Rx/Frequency and Time Synchronizer/Preamble Detector/FIFO/Validate Input Push Pop/Compare To Constant ==
  u : Inport  OutDataTypeStr=fixdt(0, 11, 0)  SampleTime=1.30208333333333e-07
  Compare : RelationalOperator  Operator===  OutDataTypeStr=boolean
  Constant : Constant  DisableCoverage=on  Value=const  OutDataTypeStr=fixdt(0, 11, 0)  SampleTime=-1
  y : Outport  SampleTime=1.30208333333333e-07
  wires:
  Compare/1 -> y/1
  Constant/1 -> Compare/2
  u/1 -> Compare/1

== system gm_commhdlQPSKTxRx/Receiver/QPSK Rx/Frequency and Time Synchronizer/Preamble Detector/FIFO/Validate Input Push Pop/Compare To Constant1 ==
  u : Inport  OutDataTypeStr=fixdt(0, 11, 0)  SampleTime=1.30208333333333e-07
  Compare : RelationalOperator  Operator===  OutDataTypeStr=boolean
  Constant : Constant  DisableCoverage=on  Value=const  OutDataTypeStr=fixdt(0, 11, 0)  SampleTime=-1
  y : Outport  SampleTime=1.30208333333333e-07
  wires:
  Compare/1 -> y/1
  Constant/1 -> Compare/2
  u/1 -> Compare/1

== system gm_commhdlQPSKTxRx/Receiver/QPSK Rx/Frequency and Time Synchronizer/Preamble Detector/FIFO/Validate Input Push Pop/MATLAB Function ==
  rst : Inport  OutDataTypeStr=boolean  PortDimensions=1  SampleTime=1.30208333333333e-07
  enb : Inport  Port=2  OutDataTypeStr=boolean  PortDimensions=1  SampleTime=1.30208333333333e-07
  dir : Inport  Port=3  OutDataTypeStr=boolean  PortDimensions=1  SampleTime=1.30208333333333e-07
  MATLAB Function : MATLAB Function  TreatAsAtomicUnit=on  mask{initVal=0, countToVal=fifoSize}
      mask prompts: initVal "Initial value:"; countToVal "Count to value:"
  count : Outport  SampleTime=1.30208333333333e-07  VectorParamsAs1DForOutWhenUnconnected=off
  wires:
  dir/1 -> MATLAB Function/3(dir)
  MATLAB Function/1(count) -> count/1
  enb/1 -> MATLAB Function/2(enb)
  rst/1 -> MATLAB Function/1(rst)

== system gm_commhdlQPSKTxRx/Receiver/QPSK Rx/Frequency and Time Synchronizer/Symbol Synchronizer/Rate Handle/FIFO/Validate Input Push Pop ==
  rst : Inport  OutDataTypeStr=boolean  PortDimensions=1  SampleTime=1.30208333333333e-07
  push : Inport  Port=2  OutDataTypeStr=boolean  PortDimensions=1  SampleTime=1.30208333333333e-07
  pop : Inport  Port=3  OutDataTypeStr=boolean  PortDimensions=1  SampleTime=1.30208333333333e-07
  Compare To Constant : Subsystem  mask(Compare To Constant){relop===, const=double(0), OutDataTypeStr=boolean, ZeroCross=on}
      mask prompts: relop "Simulink:masks:Operator_MP"; const "Simulink:masks:ConstantValue_MP"; OutDataTypeStr "Simulink:masks:OutputDataType_MP"; ZeroCross "Simulink:masks:EnableZerocrossingDetection_MP"
      mask help: Simulink:masks:CompareToConstant_MD
      mask init:
      | OutDataTypeStr = 'boolean';
      | ZeroCross = 'on';
      | blkName = 'commhdlQPSKTxRx/Receiver/QPSK Rx/Frequency and Time Synchronizer/Symbol Synchronizer/Rate Handle/FIFO/Validate Input Push Pop/Compare\nTo Constant';
      | const = double(0);
      | const_str = '0';
      | const_val = double(0);
      | relop = '==';
      | setValue = 'boolean';
      | str = '== 0';
      mask TypeOptions relop: == | ~= | < | <= | >= | >
      mask TypeOptions OutDataTypeStr: Simulink:masks:uint8 | Simulink:masks:boolean
      mask Callback ZeroCross: sl('zeroCrossEnable', gcbh);
      mask Display: disp(str)
  Compare To Constant1 : Subsystem  mask(Compare To Constant){relop===, const=double(32), OutDataTypeStr=boolean, ZeroCross=on}
      mask prompts: relop "Simulink:masks:Operator_MP"; const "Simulink:masks:ConstantValue_MP"; OutDataTypeStr "Simulink:masks:OutputDataType_MP"; ZeroCross "Simulink:masks:EnableZerocrossingDetection_MP"
      mask help: Simulink:masks:CompareToConstant_MD
      mask init:
      | OutDataTypeStr = 'boolean';
      | ZeroCross = 'on';
      | blkName = 'commhdlQPSKTxRx/Receiver/QPSK Rx/Frequency and Time Synchronizer/Symbol Synchronizer/Rate Handle/FIFO/Validate Input Push Pop/Compare\nTo Constant1';
      | const = double(32);
      | const_str = 'fifoSize';
      | const_val = [];
      | relop = '==';
      | setValue = 'boolean';
      | str = '== fifoSize';
      mask TypeOptions relop: == | ~= | < | <= | >= | >
      mask TypeOptions OutDataTypeStr: Simulink:masks:uint8 | Simulink:masks:boolean
      mask Callback ZeroCross: sl('zeroCrossEnable', gcbh);
      mask Display: disp(str)
  Constant : Constant  Value=true  OutDataTypeStr=boolean  SampleTime=-1
  Constant1 : Constant  Value=false  OutDataTypeStr=boolean  SampleTime=-1
  Delay : Delay  DelayLength=1
  Logical Operator1 : Logic  Operator=XOR  AllPortsSameDT=off  OutDataTypeStr=boolean
  Logical Operator2 : Logic  Operator=NOT  AllPortsSameDT=off  OutDataTypeStr=boolean
  Logical Operator{3..5,7,9} (5 alike) : Logic  AllPortsSameDT=off  OutDataTypeStr=boolean
  Logical Operator6 : Logic  Operator=NOT  AllPortsSameDT=off  OutDataTypeStr=boolean
  Logical Operator8 : Logic  Operator=NOT  AllPortsSameDT=off  OutDataTypeStr=boolean
  MATLAB Function : Subsystem
  Switch : Switch  Criteria=u2 ~= 0  OutDataTypeStr=boolean  SaturateOnIntegerOverflow=off  InputSameDT=off
  valid push : Outport  SampleTime=1.30208333333333e-07
  valid pop : Outport  Port=2  SampleTime=1.30208333333333e-07
  wires:
  Logical Operator3/1 -> Logical Operator6/1
  Compare To Constant1/1(y) -> Logical Operator4/2
  Logical Operator4/1 -> Logical Operator2/1
  Logical Operator6/1 -> Logical Operator7/2
  Compare To Constant/1(y) -> Logical Operator3/1
  push/1 -> Logical Operator9/1, Logical Operator5/1
  Logical Operator1/1 -> MATLAB Function/2(enb)
  Logical Operator9/1 -> valid push/1, Logical Operator1/1
  Constant1/1 -> Switch/1
  Logical Operator5/1 -> Logical Operator4/1
  pop/1 -> Logical Operator7/1, Logical Operator3/2
  MATLAB Function/1(count) -> Delay/1
  Constant/1 -> Switch/3
  Logical Operator7/1 -> valid pop/1, Logical Operator1/2, Switch/2, Logical Operator8/1
  Delay/1 -> Compare To Constant/1(u), Compare To Constant1/1(u)
  rst/1 -> MATLAB Function/1(rst)
  Switch/1 -> MATLAB Function/3(dir)
  Logical Operator8/1 -> Logical Operator5/2
  Logical Operator2/1 -> Logical Operator9/2

== system gm_commhdlQPSKTxRx/Receiver/QPSK Rx/Frequency and Time Synchronizer/Symbol Synchronizer/Rate Handle/FIFO/Validate Input Push Pop/Compare To Constant ==
  u : Inport  OutDataTypeStr=fixdt(0, 6, 0)  SampleTime=1.30208333333333e-07
  Compare : RelationalOperator  Operator===  OutDataTypeStr=boolean
  Constant : Constant  DisableCoverage=on  Value=const  OutDataTypeStr=fixdt(0, 6, 0)  SampleTime=-1
  y : Outport  SampleTime=1.30208333333333e-07
  wires:
  Compare/1 -> y/1
  Constant/1 -> Compare/2
  u/1 -> Compare/1

== system gm_commhdlQPSKTxRx/Receiver/QPSK Rx/Frequency and Time Synchronizer/Symbol Synchronizer/Rate Handle/FIFO/Validate Input Push Pop/Compare To Constant1 ==
  u : Inport  OutDataTypeStr=fixdt(0, 6, 0)  SampleTime=1.30208333333333e-07
  Compare : RelationalOperator  Operator===  OutDataTypeStr=boolean
  Constant : Constant  DisableCoverage=on  Value=const  OutDataTypeStr=fixdt(0, 6, 0)  SampleTime=-1
  y : Outport  SampleTime=1.30208333333333e-07
  wires:
  Compare/1 -> y/1
  Constant/1 -> Compare/2
  u/1 -> Compare/1

== system gm_commhdlQPSKTxRx/Receiver/QPSK Rx/Frequency and Time Synchronizer/Symbol Synchronizer/Rate Handle/FIFO/Validate Input Push Pop/MATLAB Function ==
  rst : Inport  OutDataTypeStr=boolean  PortDimensions=1  SampleTime=1.30208333333333e-07
  enb : Inport  Port=2  OutDataTypeStr=boolean  PortDimensions=1  SampleTime=1.30208333333333e-07
  dir : Inport  Port=3  OutDataTypeStr=boolean  PortDimensions=1  SampleTime=1.30208333333333e-07
  MATLAB Function : MATLAB Function  TreatAsAtomicUnit=on  mask{initVal=0, countToVal=fifoSize}
      mask prompts: initVal "Initial value:"; countToVal "Count to value:"
  count : Outport  SampleTime=1.30208333333333e-07  VectorParamsAs1DForOutWhenUnconnected=off
  wires:
  MATLAB Function/1(count) -> count/1
  dir/1 -> MATLAB Function/3(dir)
  enb/1 -> MATLAB Function/2(enb)
  rst/1 -> MATLAB Function/1(rst)

== matlab function gm_commhdlQPSKTxRx/Receiver/QPSK Rx/Frequency and Time Synchronizer/Preamble Detector/FIFO/Validate Input Push Pop/MATLAB Function/MATLAB Function ==
  data: rst input; count output; enb input; dir input; initVal parameter; countToVal parameter
function count = hdlCounter(rst,enb,dir,initVal,countToVal)
%#codegen

persistent countReg

if(isempty(countReg))
    countReg = fi(initVal,0,nextpow2(countToVal+1),0);
end

if(rst)
    countReg(:) = initVal;
elseif(enb)
    if(dir)
        if(countReg==countToVal)
            countReg(:) = initVal;
        else
            countReg(:) = countReg+1;
        end
    else
        if(countReg==initVal)
            countReg(:) = countToVal;
        else
            countReg(:) = countReg-1;
        end
    end
end

count = countReg;

end
